simulink model "applySmoothingKernel"  (R2012b)
settings: Solver=FixedStepDiscrete  StartTime=0.0  StopTime=10.0  FixedStep=0.001  RelTol=1e-3
settings Model: BufferReuse=off  Creator=gilja  LastModifiedBy=Chethan
settings SolverCC: EnableConcurrentExecution=on  ConcurrentTasks=on
settings DataIOCC: SaveOutput=off  SignalLogging=off  DSMLogging=off  SaveTime=off
settings OptimizationCC: InlineParams=on  InlineInvariantSignals=on  OptimizeBlockIOStorage=off  BufferReuse=off  ExpressionFolding=off  LocalBlockOutputs=off
settings HardwareCC: ProdIntDivRoundTo=Zero  ProdEndianess=LittleEndian  ProdHWDeviceType=Generic->32-bit x86 compatible
settings ModelReferenceCC: ModelReferenceMinAlgLoopOccurrences=on
settings RTWCC: SystemTargetFile=xpctarget.tlc  TemplateMakefile=xpc_default_tmf  Description=xPC Target  ProcessScript=xpctarget_make_rtw_hook  RTWCompilerOptimization=On
settings CodeAppCC: MaxIdLength=62
settings xpcTargetCC: TargetFcnLib=ansi_tfl_table_tmw.mat  CodeReplacementLibrary=XPC_BLAS  ParMdlRefBuildCompliant=on  ConcurrentExecutionCompliant=on  CombineSignalStateStructs=off  GRTInterface=on  xPCTaskExecutionProfile=on  xPCRL32EventNumber=5000  xPCisDownloadable=off  xPCLoadParamSetFile=off  xPCConcurrentTasks=off  xPCEnableSFAnimation=off

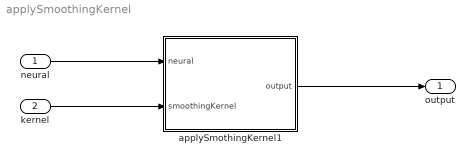
== system applySmoothingKernel ==
  neural : Inport
  kernel : Inport  Port=2
  applySmothingKernel1 : MATLAB Function  TreatAsAtomicUnit=on
  output : Outport  BusOutputAsStruct=on
  wires:
  applySmothingKernel1/1(output) -> output/1
  neural/1 -> applySmothingKernel1/1(neural)
  kernel/1 -> applySmothingKernel1/2(smoothingKernel)

== matlab function applySmoothingKernel/applySmothingKernel1 ==
  data: neural input size=[1 uint16(2*DecoderConstants.NUM_CHANNELS_PER_ARRAY)]; smoothingKernel input size=[uint16(DecoderConstants.MAX_KERNEL_LENGTH) 1]; output output
function output = applySmoothingKernel(neural, smoothingKernel)
    persistent bufferedInput
    if isempty(bufferedInput)
        bufferedInput = zeros([uint16(DecoderConstants.MAX_KERNEL_LENGTH) numel(neural) ]);
    end
    bufferedInput(2:end,:) = bufferedInput(1:end-1,:);
    
    output=zeros(1,2*uint16(DecoderConstants.NUM_CHANNELS_PER_ARRAY));

    %%% i know. it seems stupid to unroll this. but somehow the simple
    %%% matrix mult wasn't working.
    for x = coder.unroll(1:2*uint16(DecoderConstants.NUM_CHANNELS_PER_ARRAY))
        bufferedInput(1,x) = neural(x);
        output(x) = smoothingKernel(:)'*bufferedInput(:,x);
    end
